simulink model "demo_exakt_nestab"  (Simulink 2.20)
settings: Solver=ode45  StartTime=0.0  StopTime=15.0  MaxStep=0.1  RelTol=1e-3  AbsTol=1e-6
values from neighbouring files (symbols this model uses):
  v = menu('EXACT LINEARIZATION (demo simulations)',    'Exact linearization of SISO system',    'Exact linearization of MIMO system',    'System with unstable zero dynamics')    [demos_exakt.m]    (also in demos_fp.m = menu('PHASE PLANE ANALYSIS (demo simulations)',    '2nd-Orde; demos_gs.m = menu('GAIN SCHEDULING (demo simulations)',    'Input and out)
  x1 = x(j)    [fazrov_auton2.m]
  x2 = x(j+1)    [fazrov_auton2.m]    (also in fazrov_typ1.m = get_param(get_param(gcbh,'Parent'),'UserData'))
undefined symbols (not defined in the file or in its folder): x3, x4
libraries: NelinSys x4
CloseFcn:
  | ;slview('closediagram',bdroot);
settings Model: ConsistencyChecking=off  RTWPlaceOutputsASAP=off

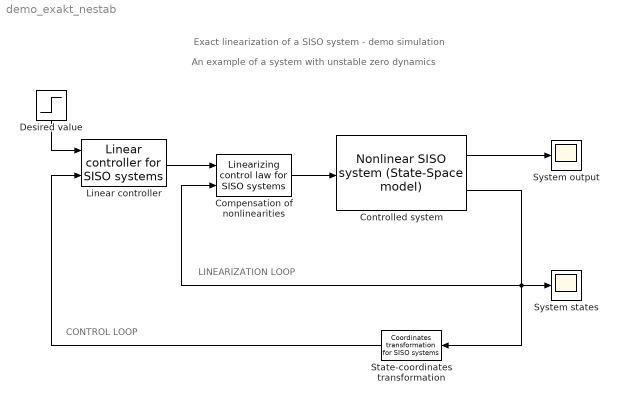
== system demo_exakt_nestab ==
  note: LINEARIZATION LOOP
  note: CONTROL LOOP
  note: Exact linearization of a SISO system - demo simulation
  note: An example of a system with unstable zero dynamics
  " Desired value" : Step  Orientation=down  Time=5  Before=2  After=10
  Compensation of nonlinearities : NelinSys/Nonlinear Systems Synthesis/Exact Linearization Blocks/Linearizing control law for SISO systems  n=4  vzorec=-1275185191261904181/1801439850948198400*sin(2*x3)-100090988508834477/1801439850948198400*x4*sin(x3)+19314281477129185/18014398509481984*v-1299882967647201/18014398509481984*v*cos(2*x3)  vzorecP=0
  Controlled system : NelinSys/Nonlinear Systems Synthesis/Nonlinear SISO system (State-Space model)  n=4  F=[x2; (1275185191261904181/900719925474099200*sin(x3)*cos(x3)+100090988508834477/1801439850948198400*x4*sin(x3))/(10307082222388193/9007199254740992-1299882967647201/9007199254740992*cos(x3)^2); x4; (-10111247660162817333/900719925474099200*sin(x3)-100090988508834477/1801439850948198400*x4*cos(x3)*sin(x3))/(793645331123890861/1801439850948198400-100090988508834477/1801439850948198400*cos(x3)^2)]  Fp=0  G=[0; 1/(10307082222388193/9007199254740992-1299882967647201/9007199254740992*cos(x3)^2); 0; -cos(x3)/(793645331123890861/1801439850948198400-100090988508834477/1801439850948198400*cos(x3)^2)]  Gp=0  H=x1  Hp=0  pp=[0 0 0 0]'
  Linear controller : NelinSys/Nonlinear Systems Synthesis/Exact Linearization Blocks/Linear controller for SISO systems  r=2  kor=[-2 -2 -6]  integ=on
  State-coordinates transformation : NelinSys/Nonlinear Systems Synthesis/Exact Linearization Blocks/Coordinates transformation for SISO systems  Orientation=left  n=4  r=2  Z=[x1; x2]  Zp=0
  System output : Scope
      settings: TickLabels=on  TimeRange=15  YMin=0  YMax=10  SaveToWorkspace=off  SaveName=ScopeData
  System states : Scope
      settings: TickLabels=on  TimeRange=15  YMin=-20  YMax=60  SaveToWorkspace=off  SaveName=ScopeData
  wires:
  Linear controller/1 -> Compensation of nonlinearities/1
  " Desired value"/1 -> Linear controller/1
  State-coordinates transformation/1 -> Linear controller/2
  Controlled system/2 -> State-coordinates transformation/1, Compensation of nonlinearities/2, System states/1
  Controlled system/1 -> System output/1
  Compensation of nonlinearities/1 -> Controlled system/1
